simulink library "rfsoc_mdl_utils"  (R2019b)
settings: Solver=VariableStepAuto  StartTime=0.0  StopTime=10.0  RelTol=1e-3
libraries: simulink x1, ddr4_behavioral_lib x1
settings Model: Creator=darenlee  LastModifiedBy=gua0154

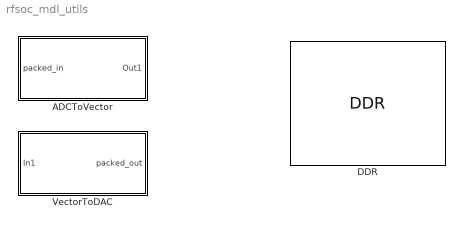
== system rfsoc_mdl_utils ==
  ADCToVector : Subsystem  mask{samplesPerClock=4, DT=fixdt(1,16,0), INPUT_DT=0}
      mask prompts: samplesPerClock "Samples Per Clock"; DT "Output Data Type"
      mask help: Convert ADC bit-concatenated input to vector outputs. Samples-per-clock will determine required input bit-width and size of the vector. Output data type will scale the data accordingly.
      mask init:
      | samplesPerClock = uint32(samplesPerClock);
      | 
      | INPUT_DT = double(16*samplesPerClock);
      mask Help: Convert ADC bit-concatenated input to vector outputs. Samples-per-clock will determine required input bit-width and size of the vector. Output data type will scale the data accordingly.
      mask DialogControl DescGroupVar Prompt: ADC Input to Vector
      mask DialogControl DescTextVar Prompt: Convert ADC bit-concatenated input to vector outputs. Samples-per-clock will determine required input bit-width and size of the vector. Output data type will scale the data accordingly.
      mask Display:
      | fprintf('ADC Input \n to Vector')
      | port_label('input',1,'ADC')
      | port_label('output',1,'Vector')
  DDR : ddr4_behavioral_lib/DDR  DDR3_DEPTH=1024  WR_RD_DATAWIDTH=128  INIT_DDR3=on  INIT_ADDR=0  INIT_DATA=fi(zeros(1,1024),0,128,0)  OutDataTypeStr=fixdt(0,128,0)  READY_DUTY_CYL=1  toggle=off
  VectorToDAC : Subsystem  mask{INPUT_WL=16, DT_INPUT=0}
      mask prompts: INPUT_WL "Shorten Input Word Length (1 to 16)"
      mask help: Take a vector of inputs and bit-concatenate the data to write to the DAC. Order of concatenation: oldest sample is the LSB and newest sample is MSB. The input word-length can be shortened prior to concatenation. Setting the shortned input wordlength to 16 will not modify the data.
      mask init:
      | if INPUT_WL <=16 && INPUT_WL >= 1 
      |     DT_INPUT = numerictype(0,INPUT_WL, INPUT_WL-1);
      | else
      |     error('Shortened input word-length must be between 1 and 16');
      | end
      mask Help: Take a vector of inputs and bit-concatenate the data to write to the DAC. Order of concatenation: oldest sample is the LSB and newest sample is MSB. The input word-length can be shortened prior to concatenation. Setting the shortned input wordlength to 16 will not modify the data.
      mask DialogControl DescGroupVar Prompt: Vector Input to DAC
      mask DialogControl DescTextVar Prompt: Take a vector of inputs and bit-concatenate the data to write to the DAC. Order of concatenation: oldest sample is the LSB and newest sample is MSB. The input word-length can be shortened prior to concatenation. Setting the shortned input wordlength to 16 will not modify the data.
      mask Display:
      | fprintf('Vector Input\n to DAC')
      | port_label('input',1,'Vector')
      | port_label('output',1,'DAC')

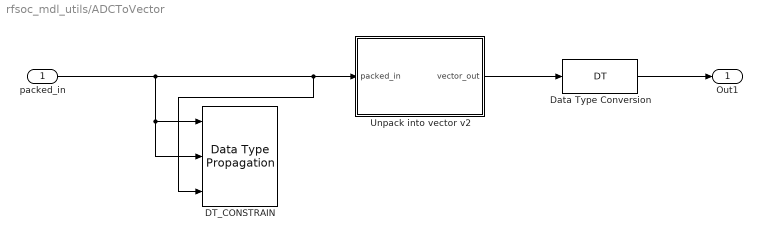
== system rfsoc_mdl_utils/ADCToVector ==
  packed_in : Inport
  DT_CONSTRAIN : simulink/Signal Attributes/Data Type Propagation  PropDataType=sfix(16)  IfRefDouble=double  IfRefSingle=double  IsSigned=IsSigned1 or IsSigned2  NumBitsBase=NumBits2  NumBitsMult=1  NumBitsAdd=0  NumBitsAllowFinal=INPUT_DT  PropScaling=2^-10  ValuesUsedBestPrec=[5 -7]  SlopeBase=Slope1  SlopeMult=1  SlopeAdd=0  BiasBase=Bias1  BiasMult=1  BiasAdd=0
      settings: SourceProductBaseCode=SL
  Data Type Conversion : DataTypeConversion  OutDataTypeStr=DT  ConvertRealWorld=Stored Integer (SI)
  Unpack into vector v2 : MATLAB Function  TreatAsAtomicUnit=on
  Out1 : Outport
  wires:
  Unpack into vector v2/1(vector_out) -> Data Type Conversion/1
  Data Type Conversion/1 -> Out1/1
  packed_in/1 -> DT_CONSTRAIN/3, Unpack into vector v2/1(packed_in), DT_CONSTRAIN/2, DT_CONSTRAIN/1

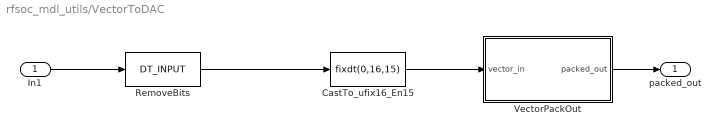
== system rfsoc_mdl_utils/VectorToDAC ==
  In1 : Inport
  CastTo_ufix16_En15 : DataTypeConversion  OutDataTypeStr=fixdt(0,16,15)  ConvertRealWorld=Stored Integer (SI)
  RemoveBits : DataTypeConversion  OutDataTypeStr=DT_INPUT  ConvertRealWorld=Stored Integer (SI)
  VectorPackOut : MATLAB Function  TreatAsAtomicUnit=on
  packed_out : Outport
  wires:
  RemoveBits/1 -> CastTo_ufix16_En15/1
  In1/1 -> RemoveBits/1
  VectorPackOut/1(packed_out) -> packed_out/1
  CastTo_ufix16_En15/1 -> VectorPackOut/1(vector_in)

== matlab function rfsoc_mdl_utils/ADCToVector/Unpack into vector v2 ==
  settings: fimath=hdlfimath
  data: packed_in input; vector_out output size=[samplesPerClock, 1]; samplesPerClock parameter size=1
function vector_out = fcn(packed_in, samplesPerClock)
%#codegen

%% Validate arguments
classes = {'int16','int32','int64','uint16','uint32','uint64','embedded.fi'};
attributes = {'size',[1 1]};
validateattributes(packed_in,classes,attributes)

classes = {'uint16','uint32','uint64','uint8'};
attributes = {'>=',1,'<=',8};
validateattributes(samplesPerClock,classes,attributes)
%%
bitsPerWord = 16;       % this is standard for RFSoC; should not change
fractionLength = 0;
outputType = numerictype(1,bitsPerWord,fractionLength);

inputLength = samplesPerClock;
unpacked_out = zeros(inputLength,1,'like',fi(0,outputType));

% Simulink seems to insist on converting fixdt(0,32,0) to uint32; convert
% it back
inputType = numerictype(0,inputLength*bitsPerWord,0);
packed_in = reinterpretcast(packed_in,inputType);

% need to unroll this loop at compile time because bitsliceget requires 
% constant inputs 
coder.unroll(); 
for n=1:inputLength
    rightIdx = (n-1)*bitsPerWord + 1;
    leftIdx  = n*bitsPerWord;
    elem =  bitsliceget(packed_in,leftIdx,rightIdx);
    unpacked_out(n) = reinterpretcast(elem, outputType);
end


vector_out = unpacked_out;

== matlab function rfsoc_mdl_utils/VectorToDAC/VectorPackOut ==
  data: vector_in input; packed_out output size=1
function packed_out = fcn(vector_in)
%#codegen

packed_out = bitconcat(vector_in(end:-1:1));
